simulink model "Vehiclemodel"  (Simulink 7.4)
settings: Solver=ode45  StartTime=0.0  StopTime=15  RelTol=1e-3
undefined symbols (not defined in the file): g, I, m, mu, Rr, slip, v0
settings Model: Creator=carlj  LastModifiedBy=alesch
settings DataIOCC: SaveOutput=off  SaveTime=off
settings OptimizationCC: InlineParams=on
settings DebuggingCC: StrictBusMsg=ErrorLevel1

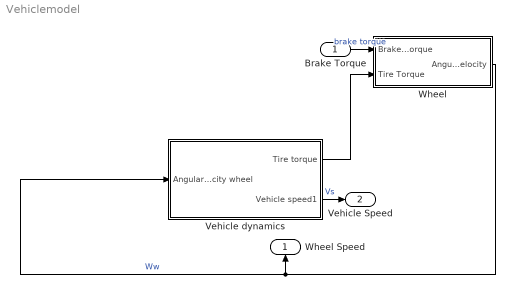
== system Vehiclemodel ==
  Brake Torque : Inport  PortDimensions=1  SampleTime=0  DataType=double  OutDataTypeStr=double
  Vehicle dynamics : Subsystem
  Wheel : Subsystem
  Wheel Speed : Outport  PortDimensions=1  SampleTime=0  DataType=double  OutDataTypeStr=double
  Vehicle Speed : Outport  Port=2  PortDimensions=1  SampleTime=0  DataType=double  OutDataTypeStr=double
  wires:
  Vehicle dynamics/2(Vehicle speed1) -> Vehicle Speed/1  "Vs"
  Brake Torque/1 -> Wheel/1(Brake Torque)  "brake torque"
  Vehicle dynamics/1(Tire torque) -> Wheel/2(Tire Torque)
  Wheel/1(Angular velocity) -> Wheel Speed/1, Vehicle dynamics/1(Angular velocity wheel)  "Ww"

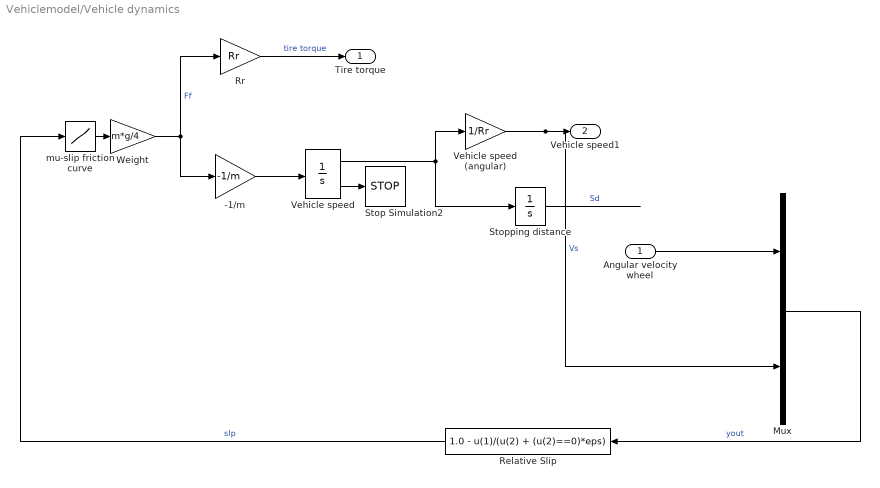
== system Vehiclemodel/Vehicle dynamics ==
  Angular velocity wheel : Inport
  -1/m : Gain  Gain=-1/m  ParameterDataType=sfix(16)  ParameterScaling=2^0  OutDataType=sfix(16)  OutScaling=2^0  SaturateOnIntegerOverflow=on  OutDataTypeStr=Inherit: Same as input  ParamDataTypeStr=Inherit: Same as input
  Mux : Mux  Inputs=2
  Relative Slip : Fcn  Expr=1.0 - u(1)/(u(2) + (u(2)==0)*eps)
  Rr : Gain  Gain=Rr  ParameterDataType=sfix(16)  ParameterScaling=2^0  OutDataType=sfix(16)  OutScaling=2^0  SaturateOnIntegerOverflow=on  OutDataTypeStr=Inherit: Same as input  ParamDataTypeStr=Inherit: Same as input
  Stop Simulation2 : Stop
  Stopping distance : Integrator  UpperSaturationLimit=1000  LowerSaturationLimit=0
  Vehicle speed : Integrator  InitialCondition=v0  LimitOutput=on  UpperSaturationLimit=1000  LowerSaturationLimit=0  ShowSaturationPort=on
  Vehicle speed (angular) : Gain  Gain=1/Rr  ParameterDataType=sfix(16)  ParameterScaling=2^0  OutDataType=sfix(16)  OutScaling=2^0  SaturateOnIntegerOverflow=on  OutDataTypeStr=Inherit: Same as input  ParamDataTypeStr=Inherit: Same as input
  Weight : Gain  Gain=m*g/4  ParameterDataType=sfix(16)  ParameterScaling=2^0  OutDataType=sfix(16)  OutScaling=2^0  SaturateOnIntegerOverflow=on  OutDataTypeStr=Inherit: Same as input  ParamDataTypeStr=Inherit: Same as input
  mu-slip friction curve : Lookup  InputValues=slip  Table=mu  OutDataType=sfix(16)  OutScaling=2^0  SaturateOnIntegerOverflow=on
  Tire torque : Outport
  Vehicle speed1 : Outport  Port=2
  wires:
  Relative Slip/1 -> mu-slip friction curve/1  "slp"
  Angular velocity wheel/1 -> Mux/1
  Mux/1 -> Relative Slip/1  "yout"
  Stopping distance/1 -> ?  "Sd"
  Vehicle speed (angular)/1 -> Mux/2, Vehicle speed1/1  "Vs"
  Rr/1 -> Tire torque/1  "tire torque"
  Weight/1 -> Rr/1, -1/m/1  "Ff"
  mu-slip friction curve/1 -> Weight/1
  Vehicle speed/1 -> Vehicle speed (angular)/1, Stopping distance/1
  Vehicle speed/2 -> Stop Simulation2/1
  -1/m/1 -> Vehicle speed/1

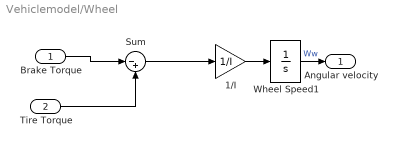
== system Vehiclemodel/Wheel ==
  Brake Torque : Inport
  Tire Torque : Inport  Port=2
  1/I : Gain  Gain=1/I  ParameterDataType=sfix(16)  ParameterScaling=2^0  OutDataType=sfix(16)  OutScaling=2^0  SaturateOnIntegerOverflow=on  OutDataTypeStr=Inherit: Same as input  ParamDataTypeStr=Inherit: Same as input
  Sum : Sum  Inputs=|-+  OutDataType=sfix(16)  OutScaling=2^0  SaturateOnIntegerOverflow=on  InputSameDT=on  OutDataTypeStr=Inherit: Same as first input
  Wheel Speed1 : Integrator  InitialCondition=v0/Rr  LimitOutput=on  UpperSaturationLimit=1000  LowerSaturationLimit=0
  Angular velocity : Outport
  wires:
  Tire Torque/1 -> Sum/2
  Sum/1 -> 1/I/1
  Brake Torque/1 -> Sum/1
  Wheel Speed1/1 -> Angular velocity/1  "Ww"
  1/I/1 -> Wheel Speed1/1
